simulink model "shiyan"  (R2016b)
settings: Solver=VariableStepAuto  StartTime=0.0  StopTime=inf  RelTol=1e-3
settings Model: Creator=11469  LastModifiedBy=11469

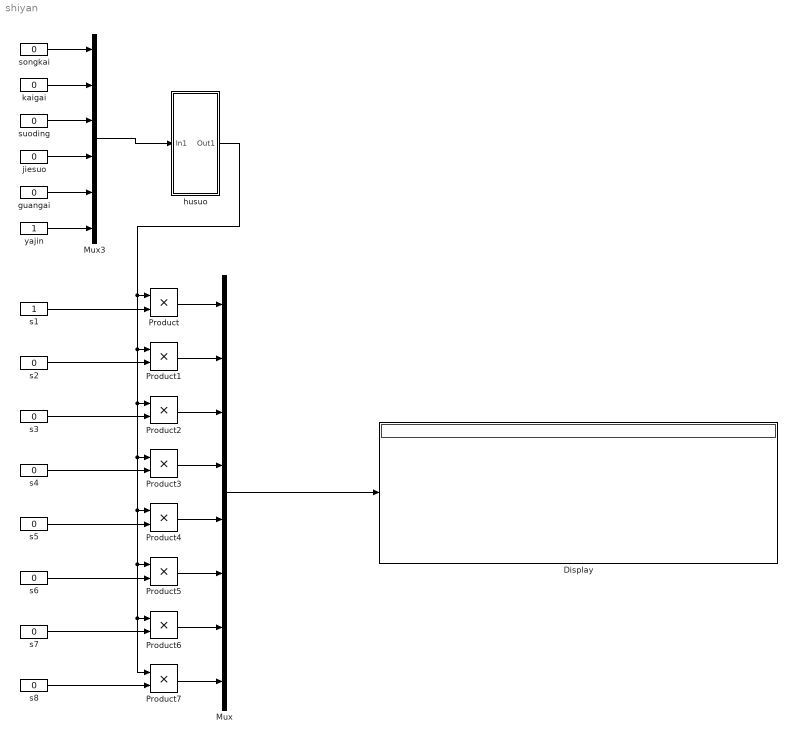
== system shiyan ==
  Display : Display
  Mux : Mux  Inputs=8
  Mux3 : Mux  Inputs=6
  Product{,1..7} (8 alike) : Product
  guangai : Constant  Value=0
      settings: OpenFcn=|
      | if get_param(gcb,'value')=='1',
      | set_param(gcb,'value','0');
      | else
      | set_param(gcb,'value','1');end
  husuo : Subsystem
  jiesuo : Constant  Value=0
      settings: OpenFcn=|
      | if get_param(gcb,'value')=='1',
      | set_param(gcb,'value','0');
      | else
      | set_param(gcb,'value','1');end
  kaigai : Constant  Value=0
      settings: OpenFcn=|
      | if get_param(gcb,'value')=='1',
      | set_param(gcb,'value','0');
      | else
      | set_param(gcb,'value','1');end
  s1 : Constant
      settings: OpenFcn=|
      | if get_param(gcb,'value')=='1',
      | set_param(gcb,'value','0');
      | else
      | set_param(gcb,'value','1');end
  s{2..8} (7 alike) : Constant  Value=0
      settings: OpenFcn=|
      | if get_param(gcb,'value')=='1',
      | set_param(gcb,'value','0');
      | else
      | set_param(gcb,'value','1');end
  songkai : Constant  Value=0
      settings: OpenFcn=|
      | if get_param(gcb,'value')=='1',
      | set_param(gcb,'value','0');
      | else
      | set_param(gcb,'value','1');end
  suoding : Constant  Value=0
      settings: OpenFcn=|
      | if get_param(gcb,'value')=='1',
      | set_param(gcb,'value','0');
      | else
      | set_param(gcb,'value','1');end
  yajin : Constant
      settings: OpenFcn=|
      | if get_param(gcb,'value')=='1',
      | set_param(gcb,'value','0');
      | else
      | set_param(gcb,'value','1');end
  wires:
  kaigai/1 -> Mux3/2
  guangai/1 -> Mux3/5
  jiesuo/1 -> Mux3/4
  songkai/1 -> Mux3/1
  yajin/1 -> Mux3/6
  suoding/1 -> Mux3/3
  Mux3/1 -> husuo/1(In1)
  s4/1 -> Product3/2
  s6/1 -> Product5/2
  s1/1 -> Product/2
  husuo/1(Out1) -> Product7/1, Product6/1, Product5/1, Product4/1, Product3/1, Product2/1, Product1/1, Product/1
  Product/1 -> Mux/1
  s2/1 -> Product1/2
  Product1/1 -> Mux/2
  s3/1 -> Product2/2
  Product2/1 -> Mux/3
  Product3/1 -> Mux/4
  Product4/1 -> Mux/5
  s5/1 -> Product4/2
  Product5/1 -> Mux/6
  Product6/1 -> Mux/7
  s7/1 -> Product6/2
  Product7/1 -> Mux/8
  s8/1 -> Product7/2
  Mux/1 -> Display/1

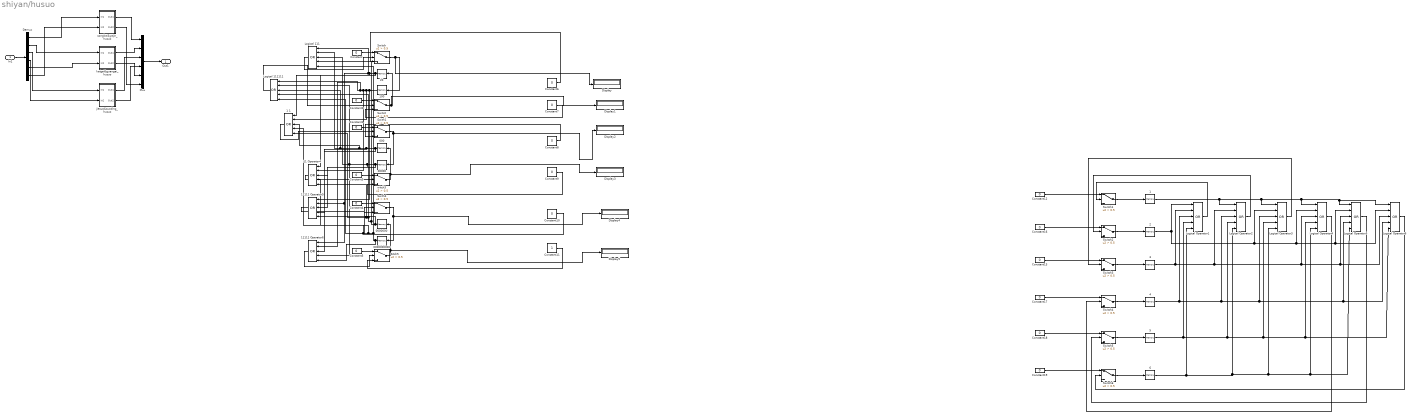
== system shiyan/husuo ==
  In1 : Inport
  000 : Memory
  00000 : Memory
  0000000 : Memory
  0000000000 : Memory
  {1..6,20,100} (8 alike) : Memory
  1 1 : Logic  Operator=OR  Inputs=5  AllPortsSameDT=off  OutDataTypeStr=boolean
  11 Operator4 : Logic  Operator=OR  Inputs=5  AllPortsSameDT=off  OutDataTypeStr=boolean
  11111 Operator5 : Logic  Operator=OR  Inputs=5  AllPortsSameDT=off  OutDataTypeStr=boolean
  11111 Operator6 : Logic  Operator=OR  Inputs=5  AllPortsSameDT=off  OutDataTypeStr=boolean
  Constant{,1..10,12..13,16..19} (17 alike) : Constant  Value=0
  Constant11 : Constant
  Demux : Demux  Outputs=6
  Display{,1..5} (6 alike) : Display
  Logical 111 : Logic  Operator=OR  Inputs=5  AllPortsSameDT=off  OutDataTypeStr=boolean
  Logical 111111 : Logic  Operator=OR  Inputs=5  AllPortsSameDT=off  OutDataTypeStr=boolean
  Logical Operator{1..6} (6 alike) : Logic  Operator=OR  Inputs=5  AllPortsSameDT=off  OutDataTypeStr=boolean
  Mux : Mux  Inputs=6
  Sitch5 : Switch  Criteria=u2 > Threshold  Threshold=0.5
  Switc2 : Switch  Criteria=u2 > Threshold  Threshold=0.5
  Switch{,1..6} (7 alike) : Switch  Criteria=u2 > Threshold  Threshold=0.5
  Swith1 : Switch  Criteria=u2 > Threshold  Threshold=0.5
  Swith4 : Switch  Criteria=u2 > Threshold  Threshold=0.5
  jiesuo&suoding_husuo : Subsystem
  kaigai&guangai_husuo : Subsystem
  songkai&yajin_husuo : Subsystem
  witch3 : Switch  Criteria=u2 > Threshold  Threshold=0.5
  Out1 : Outport
  wires:
  Demux/3 -> jiesuo&suoding_husuo/1(In1)
  Demux/4 -> jiesuo&suoding_husuo/2(In2)
  Demux/1 -> songkai&yajin_husuo/1(In1)
  songkai&yajin_husuo/1(Out1) -> Mux/1
  Demux/2 -> kaigai&guangai_husuo/1(In1)
  kaigai&guangai_husuo/1(Out1) -> Mux/2
  Demux/5 -> kaigai&guangai_husuo/2(In2)
  Demux/6 -> songkai&yajin_husuo/2(In2)
  kaigai&guangai_husuo/2(Out2) -> Mux/5
  songkai&yajin_husuo/2(Out2) -> Mux/6
  jiesuo&suoding_husuo/1(Out1) -> Mux/3
  jiesuo&suoding_husuo/2(Out2) -> Mux/4
  In1/1 -> Demux/1
  Mux/1 -> Out1/1
  Constant2/1 -> Switc2/1
  Constant/1 -> Switch/1
  Constant3/1 -> witch3/1
  Constant1/1 -> Swith1/1
  Swith1/1 -> Display2/1, 00000/1
  witch3/1 -> Display3/1, 000/1
  Constant5/1 -> Sitch5/1
  Constant4/1 -> Swith4/1
  Swith4/1 -> Display4/1, 0000000000/1
  Sitch5/1 -> Display5/1, 0000000/1
  Switch/1 -> Display/1, 100/1
  Switc2/1 -> Display1/1, 20/1
  Logical 111/1 -> Switch/2
  Logical 111111/1 -> Switc2/2
  1 1/1 -> Swith1/2
  11 Operator4/1 -> witch3/2
  11111 Operator5/1 -> Swith4/2
  11111 Operator6/1 -> Sitch5/2
  20/1 -> 11 Operator4/1, 11111 Operator6/1, 11111 Operator5/2, Logical 111/1, 1 1/1
  000/1 -> 11111 Operator6/3, 11111 Operator5/4, 1 1/3, Logical 111111/3, Logical 111/2
  00000/1 -> 11111 Operator5/3, 11 Operator4/3, 11111 Operator6/4, Logical 111111/2, Logical 111/3
  0000000/1 -> 11111 Operator5/5, 11 Operator4/5, 1 1/5, Logical 111111/4, Logical 111/4
  0000000000/1 -> 11111 Operator6/5, 11 Operator4/4, 1 1/4, Logical 111111/5, Logical 111/5
  100/1 -> 11111 Operator5/1, 1 1/2, 11 Operator4/2, 11111 Operator6/2, Logical 111111/1
  Constant6/1 -> Switch/3
  Constant7/1 -> Switc2/3
  Constant8/1 -> Swith1/3
  Constant9/1 -> witch3/3
  Constant10/1 -> Swith4/3
  Constant11/1 -> Sitch5/3
  Constant16/1 -> Switch2/1
  Constant12/1 -> Switch1/1
  Constant17/1 -> Switch4/1
  Constant13/1 -> Switch3/1
  Constant19/1 -> Switch6/1
  Constant18/1 -> Switch5/1
  Switch1/1 -> 1/1
  Switch2/1 -> 2/1
  Switch3/1 -> 3/1
  Switch4/1 -> 4/1
  Switch5/1 -> 5/1
  Switch6/1 -> 6/1
  2/1 -> Logical Operator6/2, Logical Operator5/2, Logical Operator4/2, Logical Operator3/2, Logical Operator1/1
  3/1 -> Logical Operator6/3, Logical Operator5/3, Logical Operator4/3, Logical Operator2/2, Logical Operator1/2
  4/1 -> Logical Operator6/4, Logical Operator5/4, Logical Operator3/3, Logical Operator2/3, Logical Operator1/3
  5/1 -> Logical Operator6/5, Logical Operator4/4, Logical Operator3/4, Logical Operator2/4, Logical Operator1/4
  6/1 -> Logical Operator5/5, Logical Operator4/5, Logical Operator3/5, Logical Operator2/5, Logical Operator1/5
  1/1 -> Logical Operator6/1, Logical Operator5/1, Logical Operator4/1, Logical Operator3/1, Logical Operator2/1
  Logical Operator1/1 -> Switch1/2
  Logical Operator2/1 -> Switch2/2
  Logical Operator3/1 -> Switch3/2
  Logical Operator4/1 -> Switch4/2
  Logical Operator5/1 -> Switch5/2
  Logical Operator6/1 -> Switch6/2
  ? -> Switch2/3
  ? -> Switch5/3
  ? -> Switch4/3
  ? -> Switch1/3
  ? -> Switch6/3
  ? -> Switch3/3

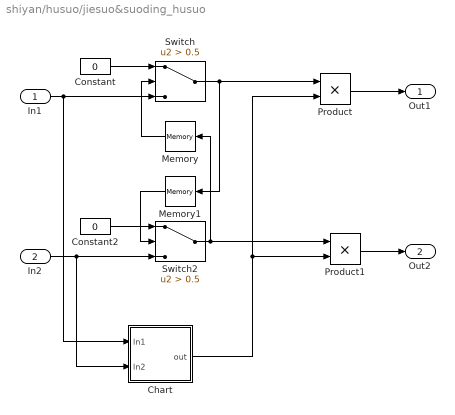
== system shiyan/husuo/jiesuo&suoding_husuo ==
  In1 : Inport
  In2 : Inport  Port=2
  Chart : Stateflow chart  TreatAsAtomicUnit=on
  Constant : Constant  Value=0
  Constant2 : Constant  Value=0
  Memory : Memory
  Memory1 : Memory
  Product : Product
  Product1 : Product
  Switch : Switch  Criteria=u2 > Threshold  Threshold=0.5
  Switch2 : Switch  Criteria=u2 > Threshold  Threshold=0.5
  Out1 : Outport
  Out2 : Outport  Port=2
  wires:
  Product1/1 -> Out2/1
  Product/1 -> Out1/1
  Chart/1(out) -> Product1/2, Product/2
  Switch2/1 -> Memory/1, Product1/1
  Constant/1 -> Switch/1
  Switch/1 -> Memory1/1, Product/1
  Constant2/1 -> Switch2/1
  In2/1 -> Switch2/3, Chart/2(ln2)
  In1/1 -> Switch/3, Chart/1(ln1)
  Memory1/1 -> Switch2/2
  Memory/1 -> Switch/2

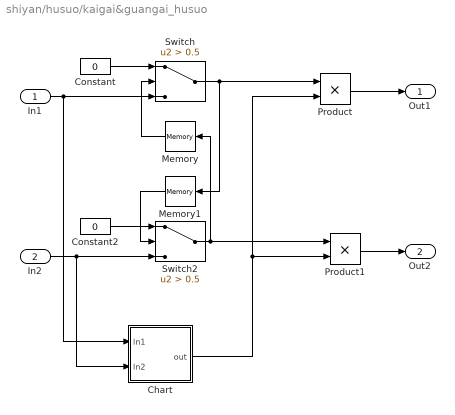
== system shiyan/husuo/kaigai&guangai_husuo ==
  In1 : Inport
  In2 : Inport  Port=2
  Chart : Stateflow chart  TreatAsAtomicUnit=on
  Constant : Constant  Value=0
  Constant2 : Constant  Value=0
  Memory : Memory
  Memory1 : Memory
  Product : Product
  Product1 : Product
  Switch : Switch  Criteria=u2 > Threshold  Threshold=0.5
  Switch2 : Switch  Criteria=u2 > Threshold  Threshold=0.5
  Out1 : Outport
  Out2 : Outport  Port=2
  wires:
  Product1/1 -> Out2/1
  Product/1 -> Out1/1
  Chart/1(out) -> Product1/2, Product/2
  Switch2/1 -> Memory/1, Product1/1
  Constant/1 -> Switch/1
  Switch/1 -> Memory1/1, Product/1
  Constant2/1 -> Switch2/1
  In2/1 -> Switch2/3, Chart/2(ln2)
  In1/1 -> Switch/3, Chart/1(ln1)
  Memory1/1 -> Switch2/2
  Memory/1 -> Switch/2

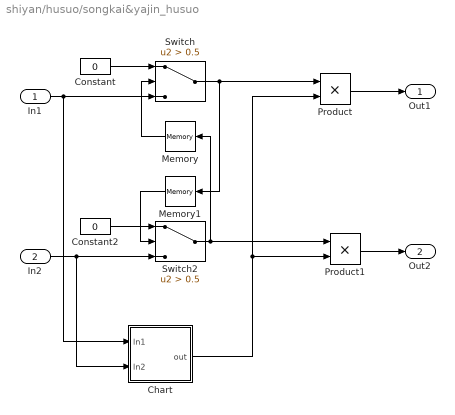
== system shiyan/husuo/songkai&yajin_husuo ==
  In1 : Inport
  In2 : Inport  Port=2
  Chart : Stateflow chart  TreatAsAtomicUnit=on
  Constant : Constant  Value=0
  Constant2 : Constant  Value=0
  Memory : Memory
  Memory1 : Memory
  Product : Product
  Product1 : Product
  Switch : Switch  Criteria=u2 > Threshold  Threshold=0.5
  Switch2 : Switch  Criteria=u2 > Threshold  Threshold=0.5
  Out1 : Outport
  Out2 : Outport  Port=2
  wires:
  Memory/1 -> Switch/2
  Memory1/1 -> Switch2/2
  In1/1 -> Chart/1(ln1), Switch/3
  In2/1 -> Chart/2(ln2), Switch2/3
  Constant2/1 -> Switch2/1
  Switch/1 -> Product/1, Memory1/1
  Constant/1 -> Switch/1
  Switch2/1 -> Product1/1, Memory/1
  Chart/1(out) -> Product/2, Product1/2
  Product/1 -> Out1/1
  Product1/1 -> Out2/1

== stateflow chart shiyan/husuo/jiesuo&suoding_husuo/Chart ==
  state A
  state A1
    en:
    out=0;
  state A2
    en:
    out=1;
  (default) -> A
  A -> (junction 3)
  (junction 3) -> A2 [order 3] : [ln1==0&&ln2==1]
  (junction 3) -> A2 [order 2] : [ln1==1&&ln2==0]
  (junction 3) -> A1 [order 1] : [ln1==1&&ln2==1]
  A1 -> A2 : [ln1==0||ln2==0]
  data: ln1 input; ln2 input; out output

== stateflow chart shiyan/husuo/kaigai&guangai_husuo/Chart ==
  state A
  state A1
    en:
    out=0;
  state A2
    en:
    out=1;
  (default) -> A
  A -> (junction 3)
  (junction 3) -> A2 [order 3] : [ln1==0&&ln2==1]
  (junction 3) -> A2 [order 2] : [ln1==1&&ln2==0]
  (junction 3) -> A1 [order 1] : [ln1==1&&ln2==1]
  A1 -> A2 : [ln1==0||ln2==0]
  data: ln1 input; ln2 input; out output

== stateflow chart shiyan/husuo/songkai&yajin_husuo/Chart ==
  state A
  state A1
    en:
    out=0;
  state A2
    en:
    out=1;
  (default) -> A
  A -> (junction 3)
  (junction 3) -> A2 [order 3] : [ln1==0&&ln2==1]
  (junction 3) -> A2 [order 2] : [ln1==1&&ln2==0]
  (junction 3) -> A1 [order 1] : [ln1==1&&ln2==1]
  A1 -> A2 : [ln1==0||ln2==0]
  data: ln1 input; ln2 input; out output
